simulink model "PV_MPPT_INV_DIST_C1"  (R2016b)
settings: Solver=VariableStepAuto  StartTime=0.0  StopTime=1  RelTol=1e-3  EnableMultiTasking=on
undefined symbols (not defined in the file): D1, Delta
libraries: powerlib x91, powerlib_meascontrol x6, re_lib x1
settings Model: Creator=Rangga  LastModifiedBy=Rangga Putra
settings OptimizationCC: LifeSpan=inf
settings DebuggingCC: SFUnexpectedBacktrackingDiag=warning  SFNoUnconditionalDefaultTransitionDiag=warning  SFExecutionAtInitializationDiag=none
settings GRTTargetCC: TargetLangStandard=C89/C90 (ANSI)  GeneratePreprocessorConditionals=Disable all
settings ConfigComp: CovMetricSettings=dw  CovHtmlReporting=on  CovSaveCumulativeToWorkspaceVar=on  CovSaveSingleToWorkspaceVar=on  CovExternalEMLEnable=off

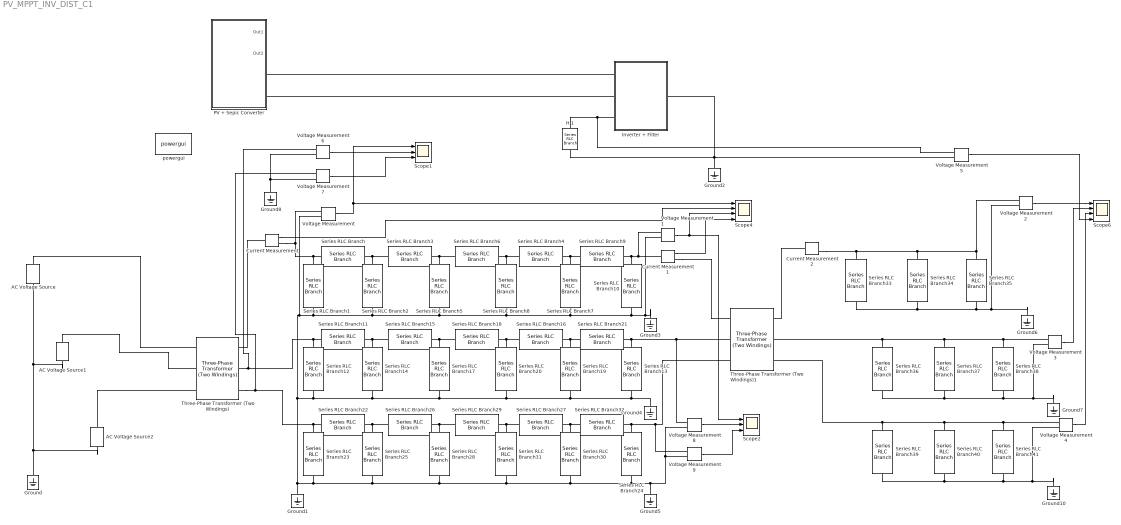
== system PV_MPPT_INV_DIST_C1 ==
  AC Voltage Source : powerlib/Electrical Sources/AC Voltage Source  Amplitude=128.1*sqrt(2)  Phase=0  Frequency=60  SampleTime=0  Measurements=None  BusType=PQ  Pref=1e3  Qref=0  Qmin=-inf  Qmax=+inf
  AC Voltage Source1 : powerlib/Electrical Sources/AC Voltage Source  Amplitude=128.7*sqrt(2)  Phase=120  Frequency=60  SampleTime=0  Measurements=None  BusType=PV  Pref=1e3  Qref=0  Qmin=-inf  Qmax=+inf
  AC Voltage Source2 : powerlib/Electrical Sources/AC Voltage Source  Amplitude=127.4*sqrt(2)  Phase=240  Frequency=60  SampleTime=0  Measurements=None  BusType=PV  Pref=1e3  Qref=0  Qmin=-inf  Qmax=+inf
  Current Measurement : powerlib/Measurements/Current Measurement  PhasorSimulation=off  OutputType=Complex  PSBequivalent=0
  Current Measurement1 : powerlib/Measurements/Current Measurement  PhasorSimulation=off  OutputType=Complex  PSBequivalent=0
  Current Measurement2 : powerlib/Measurements/Current Measurement  PhasorSimulation=off  OutputType=Complex  PSBequivalent=0
  Ground{,1..8,10} (10 alike) : powerlib/Elements/Ground  LConnTagsString=a
  H 1 : powerlib/Elements/Series RLC Branch  LConnTagsString=__new0  RConnTagsString=__new0  BranchType=RL  Resistance=2  Inductance=100e-6  SetiL0=off  InitialCurrent=0  Capacitance=1000e-6  Setx0=off  InitialVoltage=0  Measurements=None
  Inverter + Filter : Subsystem
  PV + Sepic Converter : Subsystem
  Scope1 : Scope  NumInputPorts=3
  Scope2 : Scope  NumInputPorts=3
  Scope4 : Scope  NumInputPorts=4
  Scope6 : Scope  NumInputPorts=4
  Series RLC Branch{,3..4,6,9,11,15..16,18,21..22,26..27,29,32} (15 alike) : powerlib/Elements/Series RLC Branch  LConnTagsString=__new0  RConnTagsString=__new0  BranchType=RL  Resistance=0.52  Inductance=2.5e-3  SetiL0=off  InitialCurrent=0  Capacitance=1e-6  Setx0=off  InitialVoltage=0  Measurements=None
  Series RLC Branch{1,10,12..13,23..24} (6 alike) : powerlib/Elements/Series RLC Branch  LConnTagsString=__new0  RConnTagsString=__new0  BranchType=C  Resistance=1  Inductance=1e-3  SetiL0=off  InitialCurrent=0  Capacitance=2.5e-6  Setx0=off  InitialVoltage=0  Measurements=None
  Series RLC Branch{2,5,7..8,14,17,19..20,25,28,30..31} (12 alike) : powerlib/Elements/Series RLC Branch  LConnTagsString=__new0  RConnTagsString=__new0  BranchType=C  Resistance=1  Inductance=1e-3  SetiL0=off  InitialCurrent=0  Capacitance=5e-6  Setx0=off  InitialVoltage=0  Measurements=None
  Series RLC Branch33 : powerlib/Elements/Series RLC Branch  LConnTagsString=__new0  RConnTagsString=__new0  BranchType=R  Resistance=20  Inductance=2.5e-3  SetiL0=off  InitialCurrent=0  Capacitance=1e-6  Setx0=off  InitialVoltage=0  Measurements=None
  Series RLC Branch{34..35,37..38,40..41} (6 alike) : powerlib/Elements/Series RLC Branch  LConnTagsString=__new0  RConnTagsString=__new0  BranchType=R  Resistance=2.5  Inductance=2.5e-3  SetiL0=off  InitialCurrent=0  Capacitance=1e-6  Setx0=off  InitialVoltage=0  Measurements=None
  Series RLC Branch36 : powerlib/Elements/Series RLC Branch  LConnTagsString=__new0  RConnTagsString=__new0  BranchType=R  Resistance=20  Inductance=2.5e-3  SetiL0=off  InitialCurrent=0  Capacitance=1e-6  Setx0=off  InitialVoltage=0  Measurements=None
  Series RLC Branch39 : powerlib/Elements/Series RLC Branch  LConnTagsString=__new0  RConnTagsString=__new0  BranchType=R  Resistance=20  Inductance=2.5e-3  SetiL0=off  InitialCurrent=0  Capacitance=1e-6  Setx0=off  InitialVoltage=0  Measurements=None
  Three-Phase Transformer (Two Windings) : powerlib/Elements/Three-Phase Transformer (Two Windings)  Winding1Connection=Delta (D1)  Winding2Connection=Yg  CoreType=Three single-phase transformers  SetSaturation=off  Hysteresis=off  DataFile='hysteresis'  SetInitialFlux=off  Measurements=None  UNITS=pu  NominalPower=[ 3000 , 60 ]  Winding1=[ 208 , 0.005 , 0.002 ]  Winding2=[ 208 , 0.005 , 0.002 ]  Rm=500  Lm=500  L0=0.5  Saturation=[ 0,0 ; 0.0024,1.2 ; 1.0,1.52 ]  InitialFluxes=[ 0.8 , -0.8 , 0.7 ]  MoreParameters=off  BreakLoop=off  DataType=off  TransfoNumber=1
  Three-Phase Transformer (Two Windings)1 : powerlib/Elements/Three-Phase Transformer (Two Windings)  Winding1Connection=Delta (D1)  Winding2Connection=Yg  CoreType=Three single-phase transformers  SetSaturation=off  Hysteresis=off  DataFile='hysteresis'  SetInitialFlux=off  Measurements=None  UNITS=pu  NominalPower=[ 1500 , 60 ]  Winding1=[ 208 , 0.011 , 0.016 ]  Winding2=[ 41.5 , 0.011 , 0.016 ]  Rm=500  Lm=500  L0=0.5  Saturation=[ 0,0 ; 0.0024,1.2 ; 1.0,1.52 ]  InitialFluxes=[ 0.8 , -0.8 , 0.7 ]  MoreParameters=off  BreakLoop=off  DataType=off  TransfoNumber=1
  Voltage Measurement{,1..9} (10 alike) : powerlib/Measurements/Voltage Measurement  PhasorSimulation=off  OutputType=Complex  PSBequivalent=0
  powergui : powerlib/powergui  Priority=1  SimulationMode=Discrete  SolverType=Tustin/Backward Euler (TBE)  SampleTime=1e-6  frequency=60  SPID=off  DisableSnubberDevices=off  DisableRonSwitches=off  DisableVfSwitches=off  SwTol=0  DisplayEquations=off  Interpol=off  ExternalGateDelay=off  methode=off  Ts=10  FunctionMessages=off  echomessages=off  HookPort=off  EnableUseOfTLC=off  x0status=blocks  frequencyindice=60  Pbase=100e6  ErrMax=1e-4  Iterations=50  UnitsV=kV  UnitsW=MW  buscounter=0  RestoreLinks=warning  ResistiveCurrentMeasurement=off  Frange=[0:2:500]  Ylog=off  Xlog=on  ShowGrid=off  save=off  variable=ZData  structure=0  ZoomFFT=off  StartTime=0.0  cycles=1  DisplayStyle=1  fundamental=60  FreqAxis=off  MaxFrequency=1000  frequencyindicesteady=1  RmsSteady=1  display=off
  wires:
  Voltage Measurement/1 -> Scope1/1, Scope4/1
  Voltage Measurement2/1 -> Scope6/1
  Current Measurement1/1 -> Scope4/4
  Current Measurement/1 -> Scope4/2
  Voltage Measurement1/1 -> Scope2/1, Scope4/3
  Voltage Measurement3/1 -> Scope6/2
  Voltage Measurement4/1 -> Scope6/3
  Voltage Measurement5/1 -> Scope6/4
  Voltage Measurement6/1 -> Scope1/2
  Voltage Measurement7/1 -> Scope1/3
  Voltage Measurement8/1 -> Scope2/2
  Voltage Measurement9/1 -> Scope2/3
  connections:
  Series RLC Branch17/LConn1 -- Series RLC Branch15/RConn1 -- Series RLC Branch18/LConn1
  Series RLC Branch20/LConn1 -- Series RLC Branch18/RConn1 -- Series RLC Branch16/LConn1
  Series RLC Branch19/LConn1 -- Series RLC Branch16/RConn1 -- Series RLC Branch21/LConn1
  Series RLC Branch11/LConn1 -- Voltage Measurement6/LConn1 -- Three-Phase Transformer (Two Windings)/RConn2 -- Series RLC Branch12/LConn1
  Series RLC Branch14/LConn1 -- Series RLC Branch11/RConn1 -- Series RLC Branch15/LConn1
  Series RLC Branch25/LConn1 -- Series RLC Branch22/RConn1 -- Series RLC Branch26/LConn1
  Series RLC Branch8/LConn1 -- Series RLC Branch6/RConn1 -- Series RLC Branch4/LConn1
  Series RLC Branch2/LConn1 -- Series RLC Branch/RConn1 -- Series RLC Branch3/LConn1
  Series RLC Branch5/LConn1 -- Series RLC Branch3/RConn1 -- Series RLC Branch6/LConn1
  Series RLC Branch7/LConn1 -- Series RLC Branch4/RConn1 -- Series RLC Branch9/LConn1
  Series RLC Branch28/LConn1 -- Series RLC Branch26/RConn1 -- Series RLC Branch29/LConn1
  AC Voltage Source1/LConn1 -- AC Voltage Source2/LConn1 -- Ground/LConn1 -- AC Voltage Source/LConn1
  Series RLC Branch13/LConn1 -- Three-Phase Transformer (Two Windings)1/LConn2 -- Voltage Measurement8/LConn1 -- Series RLC Branch21/RConn1
  Series RLC Branch30/LConn1 -- Series RLC Branch27/RConn1 -- Series RLC Branch32/LConn1
  Series RLC Branch22/LConn1 -- Voltage Measurement7/LConn1 -- Three-Phase Transformer (Two Windings)/RConn3 -- Series RLC Branch23/LConn1
  Series RLC Branch31/LConn1 -- Series RLC Branch29/RConn1 -- Series RLC Branch27/LConn1
  Series RLC Branch17/RConn1 -- Series RLC Branch20/RConn1 -- Ground4/LConn1 -- Series RLC Branch13/RConn1 -- Series RLC Branch19/RConn1 -- Series RLC Branch14/RConn1 -- Series RLC Branch12/RConn1 -- Voltage Measurement1/LConn2 -- Ground3/LConn1 -- Series RLC Branch10/RConn1 -- Series RLC Branch7/RConn1 -- Series RLC Branch8/RConn1 -- Series RLC Branch5/RConn1 -- Series RLC Branch2/RConn1 -- Series RLC Branch1/RConn1 -- Voltage Measurement/LConn2 -- Ground1/LConn1 -- Series RLC Branch23/RConn1 -- Series RLC Branch30/RConn1 -- Voltage Measurement9/LConn2 -- Voltage Measurement8/LConn2 -- Ground5/LConn1 -- Series RLC Branch24/RConn1 -- Series RLC Branch31/RConn1 -- Series RLC Branch28/RConn1 -- Series RLC Branch25/RConn1
  Series RLC Branch10/LConn1 -- Series RLC Branch9/RConn1 -- Voltage Measurement1/LConn1 -- Current Measurement1/LConn1
  Series RLC Branch1/LConn1 -- Series RLC Branch/LConn1 -- Voltage Measurement/LConn1 -- Current Measurement/RConn1
  Series RLC Branch24/LConn1 -- Voltage Measurement9/LConn1 -- Three-Phase Transformer (Two Windings)1/LConn3 -- Series RLC Branch32/RConn1
  Voltage Measurement2/LConn1 -- Series RLC Branch35/LConn1 -- Current Measurement2/RConn1 -- Series RLC Branch33/LConn1 -- Series RLC Branch34/LConn1
  Series RLC Branch34/RConn1 -- Series RLC Branch33/RConn1 -- Voltage Measurement2/LConn2 -- Ground6/LConn1 -- Series RLC Branch35/RConn1
  Series RLC Branch37/LConn1 -- Voltage Measurement3/LConn1 -- Series RLC Branch38/LConn1 -- Series RLC Branch36/LConn1 -- Three-Phase Transformer (Two Windings)1/RConn2
  Series RLC Branch37/RConn1 -- Series RLC Branch36/RConn1 -- Voltage Measurement3/LConn2 -- Ground7/LConn1 -- Series RLC Branch38/RConn1
  Current Measurement1/RConn1 -- Three-Phase Transformer (Two Windings)1/LConn1
  Current Measurement/LConn1 -- Three-Phase Transformer (Two Windings)/RConn1
  Current Measurement2/LConn1 -- Three-Phase Transformer (Two Windings)1/RConn1
  AC Voltage Source1/RConn1 -- Three-Phase Transformer (Two Windings)/LConn2
  AC Voltage Source/RConn1 -- Three-Phase Transformer (Two Windings)/LConn1
  AC Voltage Source2/RConn1 -- Three-Phase Transformer (Two Windings)/LConn3
  Series RLC Branch40/LConn1 -- Voltage Measurement4/LConn1 -- Series RLC Branch41/LConn1 -- Series RLC Branch39/LConn1 -- Three-Phase Transformer (Two Windings)1/RConn3
  Series RLC Branch40/RConn1 -- Series RLC Branch39/RConn1 -- Ground10/LConn1 -- Voltage Measurement4/LConn2 -- Series RLC Branch41/RConn1
  Inverter + Filter/LConn1 -- PV + Sepic Converter/RConn1
  Inverter + Filter/LConn2 -- PV + Sepic Converter/RConn2
  Voltage Measurement5/LConn2 -- H 1/RConn1 -- Inverter + Filter/RConn1 -- Ground2/LConn1
  Voltage Measurement6/LConn2 -- Voltage Measurement7/LConn2 -- Ground8/LConn1
  Inverter + Filter/LConn3 -- H 1/LConn1 -- Voltage Measurement5/LConn1

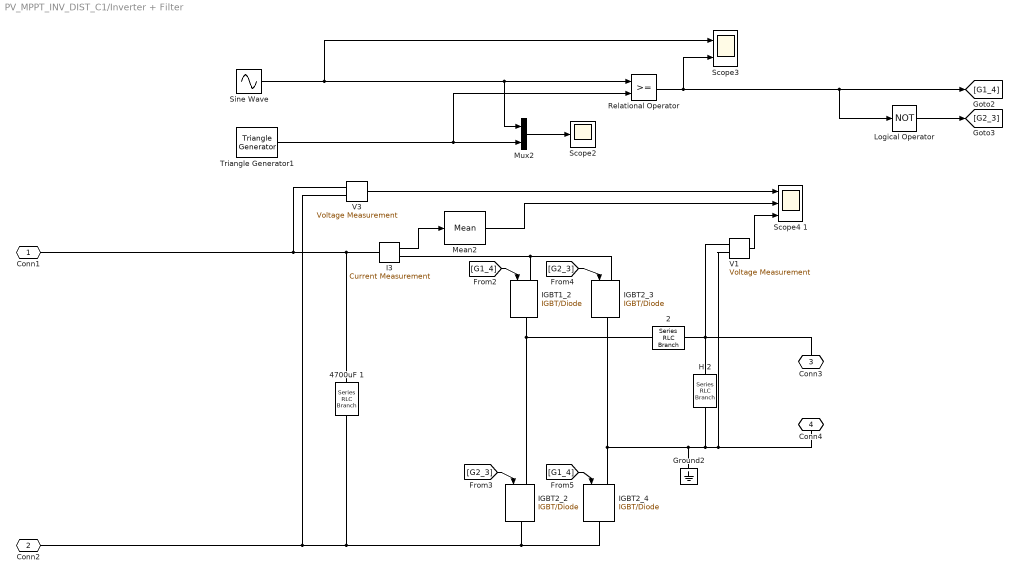
== system PV_MPPT_INV_DIST_C1/Inverter + Filter ==
  " 2" : powerlib/Elements/Series RLC Branch  LConnTagsString=__new0  RConnTagsString=__new0  BranchType=L  Resistance=3  Inductance=1500e-6  SetiL0=off  InitialCurrent=0  Capacitance=[]  Setx0=off  InitialVoltage=0  Measurements=None
  4700uF 1 : powerlib/Elements/Series RLC Branch  LConnTagsString=__new0  RConnTagsString=__new0  BranchType=C  Resistance=3  Inductance=2e-3  SetiL0=off  InitialCurrent=0  Capacitance=4700e-6  Setx0=off  InitialVoltage=0  Measurements=None
  Ground2 : powerlib/Elements/Ground  LConnTagsString=a
  H 2 : powerlib/Elements/Series RLC Branch  LConnTagsString=__new0  RConnTagsString=__new0  BranchType=C  Resistance=0.000001  Inductance=2e-3  SetiL0=off  InitialCurrent=0  Capacitance=10e-6  Setx0=off  InitialVoltage=0  Measurements=None
  I3 : powerlib/Measurements/Current Measurement  Tag=PoWeRsYsTeMmEaSuReMeNt  PhasorSimulation=off  OutputType=Magnitude  PSBequivalent=0
  IGBT1_2 : powerlib/Power Electronics/IGBT//Diode  Ron=1e-3  Rs=1e5  Cs=inf  Measurements=off
  IGBT2_2 : powerlib/Power Electronics/IGBT//Diode  Ron=1e-3  Rs=1e5  Cs=inf  Measurements=off
  IGBT2_3 : powerlib/Power Electronics/IGBT//Diode  Ron=1e-3  Rs=1e5  Cs=inf  Measurements=off
  IGBT2_4 : powerlib/Power Electronics/IGBT//Diode  Ron=1e-3  Rs=1e5  Cs=inf  Measurements=off
  Logical Operator : Logic  Operator=NOT  AllPortsSameDT=off  OutDataTypeStr=boolean
  Mean2 : powerlib_meascontrol/Measurements/Mean  Freq=60*40  Vinit=0  Ts=0
  Mux2 : Mux  Inputs=2
  Relational Operator : RelationalOperator  OutDataTypeStr=boolean  RndMeth=Nearest
  Scope2 : Scope
  Scope3 : Scope  NumInputPorts=2
  Scope4 1 : Scope  NumInputPorts=3
  Sine Wave : Sin  Amplitude=0.9  Frequency=2*pi*60  SampleTime=0
  Triangle Generator1 : powerlib_meascontrol/Pulse & Signal Generators/Triangle Generator  Freq=10000  Phase=0  Ts=0
  V1 : powerlib/Measurements/Voltage Measurement  Tag=PoWeRsYsTeMmEaSuReMeNt  PhasorSimulation=off  OutputType=Magnitude  PSBequivalent=0
  V3 : powerlib/Measurements/Voltage Measurement  Tag=PoWeRsYsTeMmEaSuReMeNt  PhasorSimulation=off  OutputType=Magnitude  PSBequivalent=0
  Conn1 : PMIOPort  Port=1  Side=Left
  Conn2 : PMIOPort  Port=2  Side=Left
  Conn3 : PMIOPort  Port=3  Side=Left
  Conn4 : PMIOPort  Port=4  Side=Right
  wires:
  I3/1 -> Mean2/1
  [G1_4] -> IGBT1_2/1
  [G2_3] -> IGBT2_2/1
  Sine Wave/1 -> Scope3/1, Relational Operator/1, Mux2/1
  V3/1 -> Scope4 1/1
  [G2_3] -> IGBT2_3/1
  [G1_4] -> IGBT2_4/1
  Relational Operator/1 -> Scope3/2, Logical Operator/1, [G1_4]
  Logical Operator/1 -> [G2_3]
  Mux2/1 -> Scope2/1
  Triangle Generator1/1 -> Mux2/2, Relational Operator/2
  Mean2/1 -> Scope4 1/2
  V1/1 -> Scope4 1/3
  connections:
  IGBT1_2/RConn1 -- " 2"/RConn1 -- IGBT2_2/LConn1
  IGBT2_4/LConn1 -- V1/LConn2 -- Conn4/RConn1 -- H 2/RConn1 -- Ground2/LConn1 -- IGBT2_3/RConn1
  IGBT2_3/LConn1 -- I3/RConn1 -- IGBT1_2/LConn1
  " 2"/LConn1 -- V1/LConn1 -- Conn3/RConn1 -- H 2/LConn1
  IGBT2_2/RConn1 -- Conn2/RConn1 -- V3/LConn2 -- 4700uF 1/RConn1 -- IGBT2_4/RConn1
  4700uF 1/LConn1 -- Conn1/RConn1 -- V3/LConn1 -- I3/LConn1

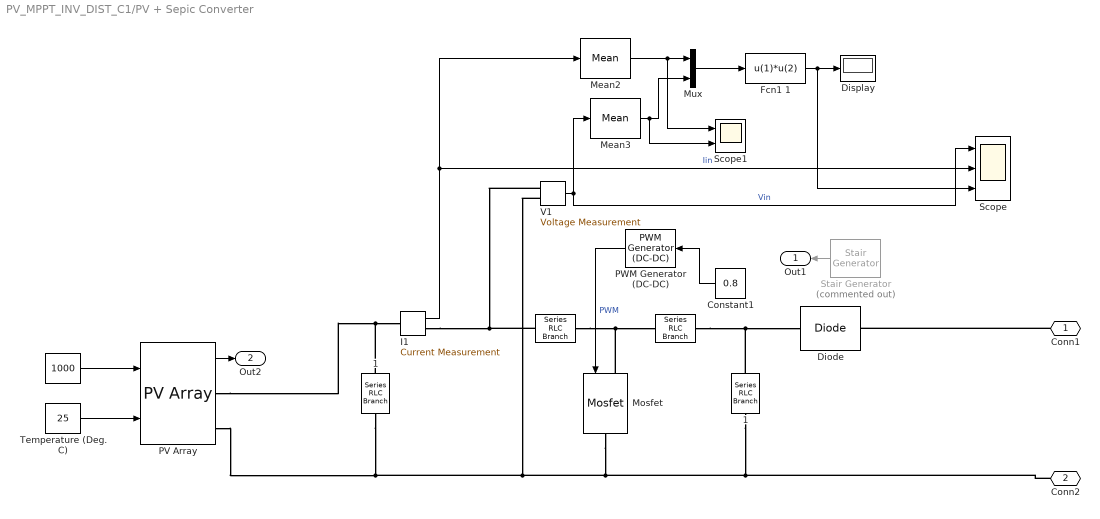
== system PV_MPPT_INV_DIST_C1/PV + Sepic Converter ==
  " " : Constant  Value=1000
  " " : powerlib/Elements/Series RLC Branch  LConnTagsString=__new0  RConnTagsString=__new0  BranchType=L  Resistance=2  Inductance=2.5e-3  SetiL0=off  InitialCurrent=0  Capacitance=[]  Setx0=off  InitialVoltage=0  Measurements=None
  " " : powerlib/Elements/Series RLC Branch  LConnTagsString=__new0  RConnTagsString=__new0  BranchType=C  Resistance=3000e-6  Inductance=2e-3  SetiL0=off  InitialCurrent=0  Capacitance=0.001  Setx0=off  InitialVoltage=10  Measurements=None
  " 1" : powerlib/Elements/Series RLC Branch  LConnTagsString=__new0  RConnTagsString=__new0  BranchType=C  Resistance=3000e-6  Inductance=2e-3  SetiL0=off  InitialCurrent=0  Capacitance=0.001  Setx0=off  InitialVoltage=10  Measurements=None
  " 1" : powerlib/Elements/Series RLC Branch  LConnTagsString=__new0  RConnTagsString=__new0  BranchType=L  Resistance=2  Inductance=1e-3  SetiL0=off  InitialCurrent=0  Capacitance=[]  Setx0=off  InitialVoltage=0  Measurements=None
  Constant1 : Constant  Value=0.8
  Diode : powerlib/Power Electronics/Diode  Ron=0.0001  Lon=0  Vf=0.8  IC=0  UseSnubber=off  Rs=0  Cs=0  Measurements=off
  Display : Display
  Fcn1 1 : Fcn  Expr=u(1)*u(2)
  I1 : powerlib/Measurements/Current Measurement  Tag=PoWeRsYsTeMmEaSuReMeNt  PhasorSimulation=off  OutputType=Magnitude  PSBequivalent=0
  Mean2 : powerlib_meascontrol/Measurements/Mean  Freq=60  Vinit=0  Ts=0
  Mean3 : powerlib_meascontrol/Measurements/Mean  Freq=60  Vinit=0  Ts=0
  Mosfet : powerlib/Power Electronics/Mosfet  Ron=0.01  Lon=0  Rd=0.01  Vfd=0  IC=0  Rs=1e5  Cs=inf  Measurements=off
  Mux : Mux  Inputs=2
  PV Array : re_lib/Solar/PV Array  Npar=1  Nser=1  PlotType=one module @ 25 deg.C & specified irradiances  S_vec=1000  Temp_C_vec=[ 45 25 100 ]  ModuleName=User-defined  PlotWhenSelected=off  Pm=99.981  Ncell=36  Voc=22.5  Isc=5.75  Vm=18.9  Im=5.29  beta_Voc_pc=-0.35  alpha_Isc_pc=0.06  beta_Voc=-0.07875  alpha_Isc=0.00345  IL=5.7591  I0=1.3543e-10  nI=0.99573  Rsh=93.7325  Rs=0.14801  BAL=on  Tc=1e-6  Tfilter=5e-5
      settings: AttributesFormatString=|
      | %<ModuleName>
      | %<Nser>-module string
      | %<Npar> parallel strings
  "PWM Generator (DC-DC) " : powerlib_meascontrol/Pulse & Signal Generators/PWM Generator (DC-DC)  Fsw=60*40  Ts=0
  Scope : Scope  NumInputPorts=3
  Scope1 : Scope  NumInputPorts=2
  Stair Generator : powerlib_meascontrol/Pulse & Signal Generators/Stair Generator  Commented=on  t=[0, 1, 2, 3, 4, 5, 6, 7, 8]  e=[0.1, 0.2, 0.3, 0.4, 0.5, 0.6, 0.7, 0.8, 0.9]  Ts=0
  Temperature (Deg. C) : Constant  Value=25
  V1 : powerlib/Measurements/Voltage Measurement  Tag=PoWeRsYsTeMmEaSuReMeNt  PhasorSimulation=off  OutputType=Magnitude  PSBequivalent=0
  Conn1 : PMIOPort  Port=1  Side=Right
  Conn2 : PMIOPort  Port=2  Side=Right
  Out1 : Outport
  Out2 : Outport  Port=2
  wires:
  "PWM Generator (DC-DC) "/1 -> Mosfet/1  "PWM"
  " "/1 -> PV Array/1
  V1/1 -> Mean3/1, Scope/1  "Vin"
  Fcn1 1/1 -> Scope/3, Display/1
  I1/1 -> Mean2/1, Scope/2  "Iin"
  Mux/1 -> Fcn1 1/1
  Mean2/1 -> Scope1/1, Mux/1
  Mean3/1 -> Scope1/2, Mux/2
  Temperature (Deg. C)/1 -> PV Array/2
  PV Array/1 -> Out2/1
  Stair Generator/1 -> Out1/1
  Constant1/1 -> "PWM Generator (DC-DC) "/1
  connections:
  " "/LConn1 -- Mosfet/LConn1 -- " "/RConn1
  " "/RConn1 -- I1/RConn1 -- V1/LConn1
  " "/LConn1 -- " 1"/RConn1 -- Diode/LConn1
  PV Array/RConn1 -- " 1"/LConn1 -- I1/LConn1
  Conn1/RConn1 -- Diode/RConn1
  " 1"/LConn1 -- Conn2/RConn1 -- Mosfet/RConn1 -- V1/LConn2 -- PV Array/RConn2 -- " 1"/RConn1
